simulink model "TWO_AREA_Load_Freq_Ctrl"  (R2021a)
settings: Solver=ode45  StartTime=0.0  StopTime=50  RelTol=1e-3  EnableMultiTasking=on
libraries: pid_lib x1
settings Model: Creator=Student  LastModifiedBy=B.HARISH
settings SolverCC: AlgebraicLoopSolver=TrustRegion
settings DataIOCC: LimitDataPoints=on  SaveFormat=Array  ReturnWorkspaceOutputs=off
settings OptimizationCC: LifeSpan=inf
settings DebuggingCC: SolverPrmCheckMsg=warning  SFUnexpectedBacktrackingDiag=warning  SFNoUnconditionalDefaultTransitionDiag=warning  SFExecutionAtInitializationDiag=none  SFMachineParentedDataDiag=warning  ArithmeticOperatorsInVariantConditions=warning
settings HardwareCC: ProdBitPerPointer=32  ProdBitPerSizeT=32  ProdBitPerPtrDiffT=32  ProdLargestAtomicFloat=None  ProdIntDivRoundTo=Undefined  ProdEndianess=Unspecified  ProdWordSize=32  ProdHWDeviceType=32-bit Generic
settings ModelReferenceCC: PropagateSignalLabelsOutOfModel=off
settings SFSimCC: SimUseLocalCustomCode=off  CustomCodeUndefinedFunction=UseInterfaceOnly
settings RTWCC: RTWUseLocalCustomCode=off
settings CodeAppCC: StateflowObjectComments=on
settings GRTTargetCC: TargetLangStandard=C89/C90 (ANSI)
settings ConfigComp: CovMetricSettings=dw  CovSaveCumulativeToWorkspaceVar=on  CovSaveSingleToWorkspaceVar=on  CovExternalEMLEnable=off  CovSFcnEnable=off

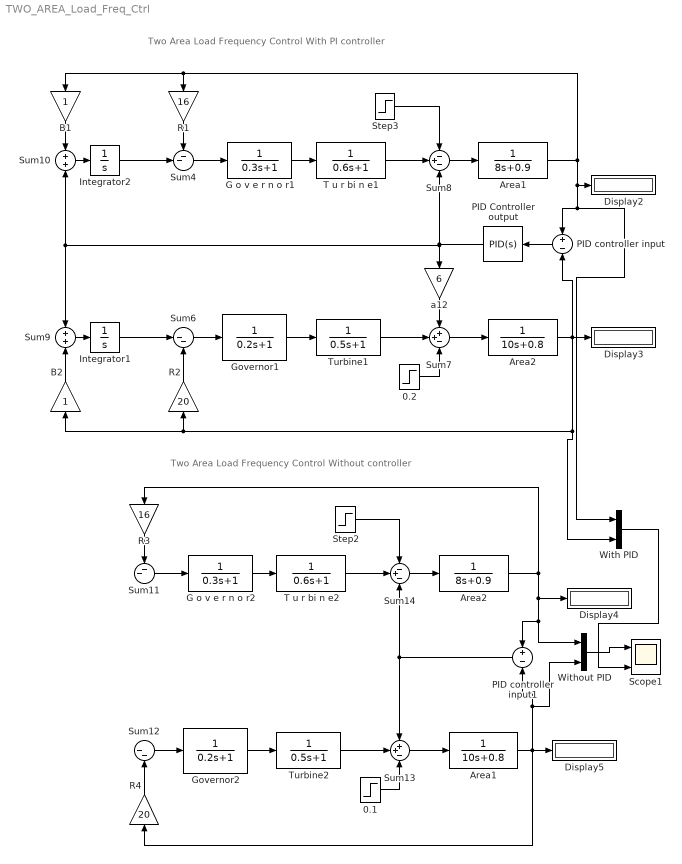
== system TWO_AREA_Load_Freq_Ctrl ==
  note: Two Area Load Frequency Control With PI controller
  note: Two Area Load Frequency Control Without controller
  "  Area1" : TransferFcn  Denominator=[8 0.9]
  "  Area2" : TransferFcn  Denominator=[8 0.9]
  " Area1" : TransferFcn  Denominator=[10 0.8]
  " Area2" : TransferFcn  Denominator=[10 0.8]
  0.1 : Step  Time=0  After=0.2  SampleTime=0
  0.2 : Step  Time=0  After=0.2  SampleTime=0
  B1 : Gain
  B2 : Gain
  Display{2..5} (4 alike) : Display
  G o v e r n o r1 : TransferFcn  Denominator=[0.3 1]  ParameterTunability=Optimized
  G o v e r n o r2 : TransferFcn  Denominator=[0.3 1]  ParameterTunability=Optimized
  Governor1 : TransferFcn  Denominator=[0.2 1]
  Governor2 : TransferFcn  Denominator=[0.2 1]
  Integrator1 : Integrator
  Integrator2 : Integrator
  PID Controller output : pid_lib/PID Controller  Controller=PID  Form=Parallel  TimeDomain=Continuous-time  UseExternalTs=off  SampleTime=-1  IntegratorMethod=Forward Euler  FilterMethod=Forward Euler  ControllerParametersSource=internal  P=5.57550599969574  I=9.98117323449892  D=0.481439807722255  UseFilter=on  N=13.7016060269838  TunerSelectOption=Transfer Function Based (PID Tuner App)  InitialConditionSource=internal  InitialConditionForIntegrator=0  InitialConditionForFilter=0  DifferentiatorICPrevScaledInput=0  ExternalReset=none  TrackingMode=off  Kt=1  LimitOutput=off  SatLimitsSource=internal  UpperSaturationLimit=inf  LowerSaturationLimit=-inf  LinearizeAsGain=on  AntiWindupMode=none  Kb=1  POutMin=[]  POutMax=[]  IOutMin=[]  IOutMax=[]  DOutMin=[]  DOutMax=[]  NOutMin=[]  NOutMax=[]  SumOutMin=[]  SumOutMax=[]  SaturationOutMin=[]  SaturationOutMax=[]  PParamMin=[]  PParamMax=[]  IParamMin=[]  IParamMax=[]  DParamMin=[]  DParamMax=[]  NParamMin=[]  NParamMax=[]  KbParamMin=[]  KbParamMax=[]  KtParamMin=[]  KtParamMax=[]  KbOutMin=[]  KbOutMax=[]  KtOutMin=[]  KtOutMax=[]  IntegratorOutMin=[]  IntegratorOutMax=[]  FilterOutMin=[]  FilterOutMax=[]  SumI1OutMin=[]  SumI1OutMax=[]  SumI2OutMin=[]  SumI2OutMax=[]  SumI3OutMin=[]  SumI3OutMax=[]  SumI4OutMin=[]  SumI4OutMax=[]  SumDOutMin=[]  SumDOutMax=[]  DifferentiatorOutMin=[]  DifferentiatorOutMax=[]  FilterDiffOutCoefMin=[]  FilterDiffOutCoefMax=[]  ReciprocalOutMin=[]  ReciprocalOutMax=[]  SumDenOutMin=[]  SumDenOutMax=[]  SumNumOutMin=[]  SumNumOutMax=[]  DivideOutMin=[]  DivideOutMax=[]  UdiffTsProdOutMin=[]  UdiffTsProdOutMax=[]  NTsProdOutMin=[]  NTsProdOutMax=[]  UintegralTsProdOutMin=[]  UintegralTsProdOutMax=[]  UngainTsProdOutMin=[]  UngainTsProdOutMax=[]  IntegratorContinuousStateAttributes=''  IntegratorStateMustResolveToSignalObject=off  IntegratorRTWStateStorageClass=Auto  FilterContinuousStateAttributes=''  FilterStateMustResolveToSignalObject=off  FilterRTWStateStorageClass=Auto  ParallelPVariant=InternalParameters  IdealPVariant=Disabled  IVariant=InternalParameters  DVariant=InternalParameters  IntegratorVariant=Continuous  SatVariant=Disabled  AWVariant=Passthrough  PCopyVariant=Disabled  TRVariant=Disabled  FdbkBlocksVariant=Forward  IdealPFdbkVariant=Disabled  SatFdbkVariant=Disabled  DerivativeFilterVariant=ContFilter  NVariant=InternalParameters  NCopyVariant=Disabled  FilterICVariant=InternalICsFilter  IntegratorICVariant=InternalICs  ExternalResetVariant=Disabled  TRSumVariant=Passthrough  SumFdbkVariant=Disabled  SumVariant=Sum_PID  TsampFilterVariant=InternalTs  TsampNgainVariant=Passthrough  TsampIntegralVariant=Passthrough  ExternalSaturationOutDataTypeStr=Inherit: Same as second input
  PID controller input : Sum  Inputs=+-
  PID controller input1 : Sum  Inputs=+-
  R1 : Gain  Gain=16
  R2 : Gain  Gain=20
  R3 : Gain  Gain=16
  R4 : Gain  Gain=20
  Scope1 : Scope  NumInputPorts=2
  Step2 : Step  Time=0  After=0.2  SampleTime=0
  Step3 : Step  Time=0  After=0.2  SampleTime=0
  Sum10 : Sum
  Sum11 : Sum  Inputs=--|
  Sum12 : Sum  Inputs=|--
  Sum13 : Sum  Inputs=++-
  Sum14 : Sum  Inputs=-+-
  Sum4 : Sum  Inputs=--|
  Sum6 : Sum  Inputs=|--
  Sum7 : Sum  Inputs=++-
  Sum8 : Sum  Inputs=-+-
  Sum9 : Sum
  T u r bi n e1 : TransferFcn  Denominator=[0.6 1]
  T u r bi n e2 : TransferFcn  Denominator=[0.6 1]
  Turbine1 : TransferFcn  Denominator=[0.5 1]
  Turbine2 : TransferFcn  Denominator=[0.5 1]
  With PID : Mux  Inputs=2
  Without PID : Mux  Inputs=2
  a12 : Gain  Gain=6
  wires:
  G o v e r n o r1/1 -> T u r bi n e1/1
  Sum6/1 -> Governor1/1
  Turbine1/1 -> Sum7/2
  R1/1 -> Sum4/1
  Sum9/1 -> Integrator1/1
  Sum8/1 -> "  Area1"/1
  B1/1 -> Sum10/1
  Governor1/1 -> Turbine1/1
  Sum7/1 -> " Area2"/1
  T u r bi n e1/1 -> Sum8/2
  "  Area1"/1 -> PID controller input/1, With PID/1, Display2/1, B1/1, R1/1
  Sum10/1 -> Integrator2/1
  " Area2"/1 -> With PID/2, B2/1, R2/1, PID controller input/2, Display3/1
  R2/1 -> Sum6/2
  B2/1 -> Sum9/2
  a12/1 -> Sum7/1
  Sum4/1 -> G o v e r n o r1/1
  Step3/1 -> Sum8/1
  0.2/1 -> Sum7/3
  PID controller input/1 -> PID Controller output/1
  PID Controller output/1 -> Sum10/2, Sum9/1, a12/1, Sum8/3
  Integrator2/1 -> Sum4/2
  Integrator1/1 -> Sum6/1
  Turbine2/1 -> Sum13/2
  Sum11/1 -> G o v e r n o r2/1
  Governor2/1 -> Turbine2/1
  Step2/1 -> Sum14/1
  R4/1 -> Sum12/2
  T u r bi n e2/1 -> Sum14/2
  Sum14/1 -> "  Area2"/1
  Sum13/1 -> " Area1"/1
  G o v e r n o r2/1 -> T u r bi n e2/1
  R3/1 -> Sum11/1
  Sum12/1 -> Governor2/1
  0.1/1 -> Sum13/3
  PID controller input1/1 -> Sum13/1, Sum14/3
  " Area1"/1 -> R4/1, Display5/1, PID controller input1/2, Without PID/2
  "  Area2"/1 -> Without PID/1, PID controller input1/1, Display4/1, R3/1
  Without PID/1 -> Scope1/1
  With PID/1 -> Scope1/2
